simulink model "Adaptive_Back_Stepping_RR"  (R2019b)
settings: Solver=VariableStepAuto  StartTime=0.0  StopTime=20  FixedStep=1e-2  RelTol=1e-3
values from neighbouring files (symbols this model uses):
  a = l1+l2*cos_q2    [Inverse_Kinematics.m]    (also in Visual.m = 0.4881; rr_planar_dynamics.m = 0.4)
  A = 0.9972    [Visual.m]    (also in rr_planar_dynamics.m = 0.5)
  B = 1.0044    [Visual.m]    (also in rr_planar_dynamics.m = 1)
  b = l2*sin_q2    [Inverse_Kinematics.m]    (also in Visual.m = 0.223; rr_planar_dynamics.m = 0.8)
  delta = 1.0436    [Visual.m]    (also in rr_planar_dynamics.m = 0.5236)
  pi_hat_0 = pi_param*(1+0.01)    [Visual.m]    (also in rr_planar_dynamics.m = pi_param*(1+0.02))
  pi_param = [0.5000; 0.1667; 0.5000; 0.1667]    [Visual.m]    (also in rr_planar_dynamics.m = [1.0000;-0.5000;0.3333;1.0000;-0.5000;0.3333])
settings Model: Creator=Stefano  LastModifiedBy=Mardok

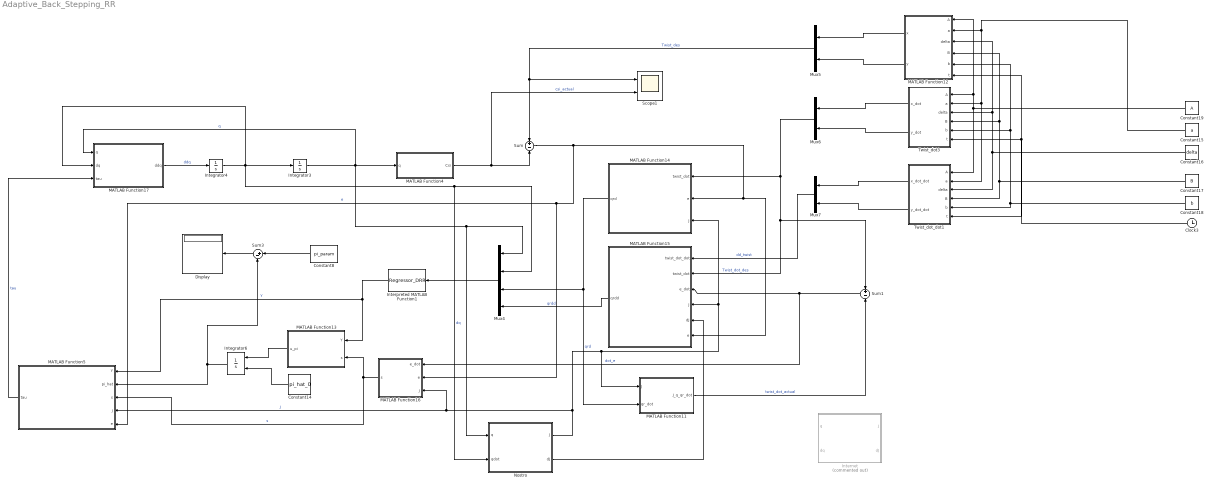
== system Adaptive_Back_Stepping_RR ==
  Clock3 : Clock
  Constant14 : Constant  Value=pi_hat_0  VectorParams1D=off
  Constant15 : Constant  Value=a
  Constant16 : Constant  Value=delta
  Constant17 : Constant  Value=B
  Constant18 : Constant  Value=b
  Constant19 : Constant  Value=A
  Constant8 : Constant  Value=pi_param
  Display : Display
  Integrator3 : Integrator  InitialCondition=[0.97,0.97]'
  Integrator4 : Integrator  InitialCondition=[0.3,0.3]'
  Integrator6 : Integrator  InitialConditionSource=external  InitialCondition=pi_hat_0
  "Internet " : MATLAB Function  Commented=on  TreatAsAtomicUnit=on
  Interpreted MATLAB Function1 : MATLABFcn  MATLABFcn=Regressor_DRR  OutputDimensions=[2,4]  Output1D=off
  MATLAB Function11 : MATLAB Function  TreatAsAtomicUnit=on
  MATLAB Function12 : MATLAB Function  TreatAsAtomicUnit=on
  MATLAB Function13 : MATLAB Function  TreatAsAtomicUnit=on
  MATLAB Function14 : MATLAB Function  TreatAsAtomicUnit=on
  MATLAB Function15 : MATLAB Function  TreatAsAtomicUnit=on
  MATLAB Function16 : MATLAB Function  TreatAsAtomicUnit=on
  MATLAB Function17 : MATLAB Function  TreatAsAtomicUnit=on
  MATLAB Function4 : MATLAB Function  TreatAsAtomicUnit=on
  MATLAB Function5 : MATLAB Function  TreatAsAtomicUnit=on
  Mux4 : Mux
  Mux5 : Mux  Inputs=2
  Mux6 : Mux  Inputs=2
  Mux7 : Mux  Inputs=2
  "Nostro " : MATLAB Function  TreatAsAtomicUnit=on
  Scope1 : Scope  NumInputPorts=2
  Sum : Sum  Inputs=+-
  Sum1 : Sum  Inputs=+-
  Sum3 : Sum  Inputs=|+-
  Twist_dot3 : MATLAB Function  TreatAsAtomicUnit=on
  Twist_dot_dot1 : MATLAB Function  TreatAsAtomicUnit=on
  wires:
  Twist_dot3/2(y_dot) -> Mux6/2
  MATLAB Function12/2(y) -> Mux5/2
  Mux4/1 -> Interpreted MATLAB Function1/1
  Twist_dot_dot1/1(x_dot_dot) -> Mux7/1
  MATLAB Function12/1(x) -> Mux5/1
  Constant14/1 -> Integrator6/2
  Twist_dot3/1(x_dot) -> Mux6/1
  Twist_dot_dot1/2(y_dot_dot) -> Mux7/2
  MATLAB Function17/1(ddq) -> Integrator4/1  "ddq"
  MATLAB Function13/1(u_pi) -> Integrator6/1
  Integrator4/1 -> MATLAB Function17/2(dq), "Nostro "/2(qdot), Mux4/2, Integrator3/1  "dq"
  Integrator3/1 -> Mux4/1, "Nostro "/1(q), MATLAB Function4/1(q), MATLAB Function17/1(q)  "q"
  MATLAB Function14/1(qrd) -> MATLAB Function11/2(qr_dot), Mux4/3  "qrd"
  MATLAB Function15/1(qrdd) -> Mux4/4  "qrdd"
  Mux6/1 -> MATLAB Function15/2(twist_dot), Sum1/1, MATLAB Function14/1(twist_dot)  "Twist_dot_des"
  MATLAB Function4/1(Csi) -> Scope1/2, Sum/2  "csi_actual"
  Mux5/1 -> Scope1/1, Sum/1  "Twist_des"
  Sum/1 -> MATLAB Function14/2(e), MATLAB Function15/6(e), MATLAB Function5/5(e), MATLAB Function16/2(e)  "e"
  "Nostro "/1(J) -> MATLAB Function15/4(J), MATLAB Function14/3(J), MATLAB Function11/1(J), MATLAB Function5/4(J), MATLAB Function16/3(J)  "J"
  Mux7/1 -> MATLAB Function15/1(twist_dot_dot)  "dd_twist"
  Sum1/1 -> MATLAB Function16/1(e_dot), MATLAB Function15/3(e_dot)  "dot_e"
  MATLAB Function11/1(J_q_qr_dot) -> Sum1/2  "twist_dot_actual"
  Interpreted MATLAB Function1/1 -> MATLAB Function5/1(Y), MATLAB Function13/1(Y)  "Y"
  MATLAB Function16/1(s) -> MATLAB Function5/3(s), MATLAB Function13/2(s)  "s"
  MATLAB Function5/1(tau) -> MATLAB Function17/3(tau)  "tau"
  Sum3/1 -> Display/1
  Clock3/1 -> Twist_dot3/6(t), Twist_dot_dot1/6(t), MATLAB Function12/6(t)
  Constant18/1 -> Twist_dot_dot1/5(b), Twist_dot3/5(b), MATLAB Function12/5(b)
  Constant17/1 -> Twist_dot_dot1/4(B), Twist_dot3/4(B), MATLAB Function12/4(B)
  Constant16/1 -> Twist_dot_dot1/3(delta), Twist_dot3/3(delta), MATLAB Function12/3(delta)
  Constant15/1 -> Twist_dot3/2(a), Twist_dot_dot1/2(a), MATLAB Function12/2(a)
  Constant19/1 -> Twist_dot_dot1/1(A), Twist_dot3/1(A), MATLAB Function12/1(A)
  Constant8/1 -> Sum3/1
  Integrator6/1 -> MATLAB Function5/2(pi_hat), Sum3/2
  "Nostro "/2(dJ) -> MATLAB Function15/5(dJ)

== matlab function Adaptive_Back_Stepping_RR/MATLAB Function11 ==
  data: J input; J_q_qr_dot output size=[2 1]; qr_dot input
function J_q_qr_dot = fcn(J,qr_dot)

J_q_qr_dot = J*qr_dot;

end

== matlab function Adaptive_Back_Stepping_RR/MATLAB Function12 ==
  data: x output; A input; y output; a input; delta input; B input; b input; t input
function [x,y] = Lissajous(A,a,delta,B,b,t)


x = A*sin(a*t+delta);
y = B*sin(b*t);


end

== matlab function Adaptive_Back_Stepping_RR/MATLAB Function13 ==
  data: Y input; u_pi output; s input
function u_pi = Update_Law(Y,s)

R = 5*ones(2,4);

u_pi = pinv(R).*(Y.')*s;
end

== matlab function Adaptive_Back_Stepping_RR/MATLAB Function14 ==
  data: twist_dot input; qrd output; e input; J input
function qrd = q_r_dot(twist_dot,e,J)

lambda = 5 * eye(2);
qrd = pinv(J)*(twist_dot + lambda * e);

end

== matlab function Adaptive_Back_Stepping_RR/MATLAB Function15 ==
  data: twist_dot_dot input; twist_dot input; qrdd output; e_dot input; J input; dJ input; e input
function qrdd = q_r_dot_dot(twist_dot_dot, twist_dot,e_dot,J,dJ,e)

lambda = 5 * eye(2);
qrdd = pinv(J)*(twist_dot_dot + lambda * e_dot) + pinv(dJ)*(twist_dot + lambda*e);
% qrdd = twist_dot_dot - lambda*e_dot;

end

== matlab function Adaptive_Back_Stepping_RR/MATLAB Function4 ==
  data: q input; Csi output
function Csi  = Direct_Kinematics_RR(q)

%INPUT: q(1) = q1;
%       q(2) = q2;

%OUTPUT: px = position along x axis
%        py = position along y axis

%Link's lenght

l1 = 1;
l2 = 0.5;

px = l1 * cos(q(1)) + l2 * cos(q(1)+q(2));
py = l1 * sin(q(1)) + l2 * sin(q(1)+q(2));

Csi = [px; py];
end

== matlab function Adaptive_Back_Stepping_RR/MATLAB Function5 ==
  data: Y input; tau output; pi_hat input; s input; J input; e input
function tau = Back_Stepping_Control_Law(Y,pi_hat,s,J,e)

Kd = 10 * eye(2);


tau = Y*pi_hat + Kd*s + (J.')*e;

end

== matlab function Adaptive_Back_Stepping_RR/MATLAB Function16 ==
  data: e_dot input; s output; e input; J input
function s = fcn(e_dot,e,J)

lamda = 5*eye(2);

s = pinv(J)*(e_dot + lamda*e);

end

== matlab function Adaptive_Back_Stepping_RR/MATLAB Function17 ==
  data: q input; ddq output; dq input; tau input
function ddq = RR_Dynamics(q,dq,tau)

% Masses
m1 = 0.5;
m2 = 0.5;
%length of the links
a1 = 1;
a2 = 0.5;
%Position of the center of mass
l1 = 0.5;
l2 = 0.25;

r1 = m1*a1*(a1-l1); %pi_primoordine_numero del link
r2 = m2*a2*(a2-l2);

% Moment Second Order
I1 = (m1*r1^2)/12;
I2 = (m2*r2^2)/12;

%Inertia matrix 
b11 = I1 + m1*l1^2 + I2 + m2*(a1^2 +l2^2 + 2*a1*l2*cos(q(2)));
b12 = I2 + m2*(l2^2 + a1*l2*cos(q(2)));
b21 = I2 + m2*(l2^2 + a1*l2*cos(q(2)));
b22 = I2 + m2*l2^2;

B = [b11,b12;
    b21,b22];

%Coriolis matrix
h = - m2*a1*l2*sin(q(2));

C = [h*dq(2), h*(dq(1)+dq(2)); 
    -h*(dq(1)), 0];

ddq = pinv(B)*(tau - C*dq);

== matlab function Adaptive_Back_Stepping_RR/Nostro  ==
  data: q input; J output; qdot input; dJ output
function [J,dJ] = Jacobian(q,qdot)

l1=1;
l2=0.5;

J = [-l1*sin(q(1))-l2*sin(q(1)+q(2)), -l2*sin(q(1)+q(2));
    l1*cos(q(1))+l2*cos(q(1)+q(2)), l2*cos(q(1)+q(2))];

dJ_11 = -l1*cos(q(1))*qdot(1) - l2*cos(q(1)+q(2))*(qdot(1)+qdot(2));
dJ_12 = -l2*cos(q(1)+q(2))*(qdot(1)+qdot(2));
dJ_21 = -l1*sin(q(1))*qdot(1)-l2*sin(q(1)+q(2))*(qdot(1)+qdot(2));
dJ_22 = -l2*sin(q(1)+q(2))*(qdot(1)+qdot(2));

dJ = [dJ_11, dJ_12; 
    dJ_21, dJ_22];

end

== matlab function Adaptive_Back_Stepping_RR/Internet  ==
  data: q input; J output; dJ output; dq input
function [J,dJ] = Jacobian(q,dq)

%v = J(q) * dq

%length of the links
l1 = 0.5;
l2 = 0.5;
%Position of the center of mass
a1 = 1;
a2 = 1;

J = [-l1*sin(q(1)), 0, -a1*sin(q(1))-l2*sin(q(1)+q(2)), -l2*sin(q(1)+q(2));
    l1*cos(q(1)), 0, a1*cos(q(1))+l2*cos(q(1)+q(2)), l2*cos(q(1)+q(2))];


dJ = zeros(2,2);

dJ_11 = -l1*cos(q(1))*dq(1);
dJ_12 = 0;
dJ_13 = -a1*cos(q(1))*dq(1)-l2*cos(q(1)+q(2))*(dq(1)+dq(2));
dJ_14 = -l2*cos(q(1)+q(2))*(dq(1)+dq(2));
dJ_21 = -l1*sin(q(1))*dq(1);
dJ_22 = 0;
dJ_23 = -a1*sin(q(1))*dq(1)-l2*sin(q(1)+q(2))*(dq(1)+dq(2));
dJ_24 = -l2*sin(q(1)+q(2))*(dq(1)+dq(2));


dJ = [dJ_11, dJ_12, dJ_13, dJ_14; 
    dJ_21, dJ_22,dJ_23, dJ_24];


end

== matlab function Adaptive_Back_Stepping_RR/Twist_dot3 ==
  data: A input; x_dot output; a input; delta input; B input; b input; t input; y_dot output
function [x_dot,y_dot] = Lissajous(A,a,delta,B,b,t)


% x = A*sin(a*t+delta);
% y = B*sin(b*t);

x_dot = A * cos(a*t + delta) * a;
y_dot = B * cos(b*t) * b;


end

== matlab function Adaptive_Back_Stepping_RR/Twist_dot_dot1 ==
  data: A input; x_dot_dot output; a input; delta input; B input; b input; t input; y_dot_dot output
function [x_dot_dot,y_dot_dot] = Lissajous(A,a,delta,B,b,t)


% x = A*sin(a*t+delta);
% y = B*sin(b*t);

x_dot_dot = -A * sin(a*t + delta) * a^2;
y_dot_dot = -B * sin(b*t) * b^2;


end
